simulink model "sysgenDWT"  (Simulink 7.0)
settings: Solver=ode45  StartTime=0.0  StopTime=4096+1024+100  RelTol=1e-3
PreLoadFcn:
  | xlrequire('imageData.mat'); xlrequire('PreLoadFcn');
PostLoadFcn:
  | open_system('sysgenDWT/Processor/Memory Controller','force'); pause(0.50); open_system('sysgenDWT');pause(0.50); close_system('sysgenDWT/Processor/Memory Controller');pause(0.50); close_system('sysgenDWT/Processor');
StopFcn:
  | xlrequire('StopFcn');
values from neighbouring files (symbols this model uses):
  b1Init = sysgenDWT_imageData( stride + dither )    [sysgenDWT_PreLoadFcn.m]
  b2Init = sysgenDWT_imageData( stride + not(dither) )    [sysgenDWT_PreLoadFcn.m]
libraries: xbsIndex_r4 x214, dspindex x4, dspmtrx3 x4, dspsnks4 x3, xbsCopyrightNotice_r4 x1, dspsrcs4 x1
(part 1 of 3)
settings Model: Creator=alexc  LastModifiedBy=douangp
settings DataIOCC: SignalLoggingName=sigsOut
settings OptimizationCC: BlockReduction=off  BooleanDataType=off  InlineInvariantSignals=on
settings DebuggingCC: SaveWithParameterizedLinksMsg=none  SignalResolutionControl=TryResolveAllWithWarning  SolverPrmCheckMsg=none  MultiTaskDSMMsg=warning  MultiTaskCondExecSysMsg=none  StrictBusMsg=None
settings HardwareCC: TargetUnknown=on
settings RTWCC: IncludeERTFirstTime=on
settings GRTTargetCC: TargetFcnLib=ansi_tfl_tmw.mat

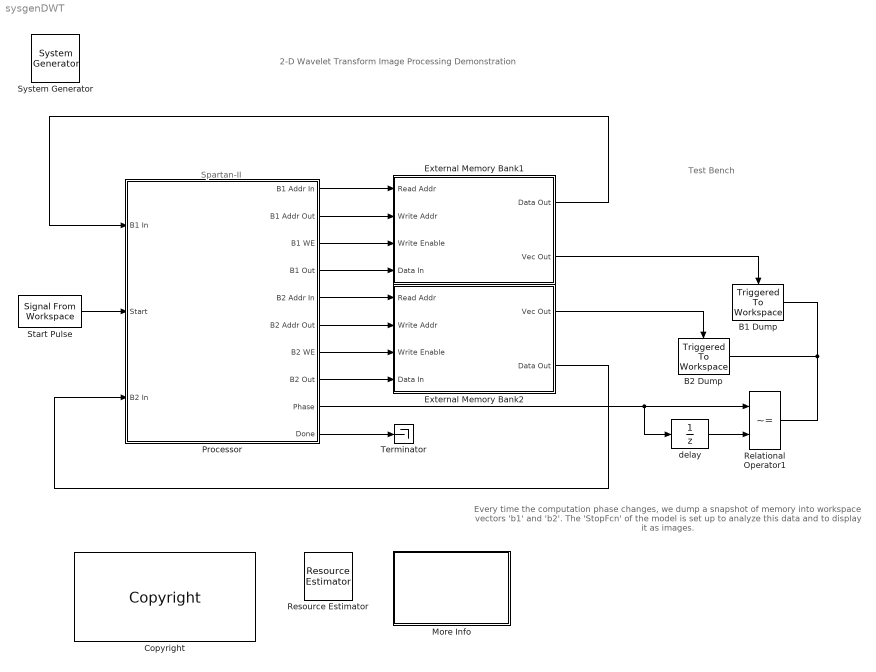
== system sysgenDWT ==
  note: Spartan-II
  note: Test
      |  Bench
  note: Every time the computation phase
      | changes, we dump a snapshot of
      | memory into workspace vectors  'b1'
      | and  'b2'.
      |
      | The 'StopFcn' of the model is set up
      | to analyze this data and to display
      | it as images.
  note: 2-D Wavelet Transform
      |  Image Processing Demonstration
  " System Generator" : xbsIndex_r4/ System Generator  Tag=genX  SystemSampleTime=-1  xilinxfamily=spartan3adsp  part=xc3sd3400a  speed=-4  package=fg676  synthesis_tool=XST  clock_wrapper=Clock Enables  directory=./netlist  testbench=off  simulink_period=1  sysclk_period=6  dcm_input_clock_period=100  incr_netlist=off  trim_vbits=Everywhere in SubSystem  dbl_ovrd=According to Block Masks  core_generation=Not Needed - Already Generated  run_coregen=off  deprecated_control=off  eval_field=0  block_type=sysgen
      settings: block_version=10.1.3
  B1 Dump : dspsnks4/Triggered To Workspace  Orientation=down  SystemSampleTime=-1  TriggerType=Falling edge  VariableName=b1  Buffer=1000
      settings: FixptAsFi=off
  B2 Dump : dspsnks4/Triggered To Workspace  Orientation=down  SystemSampleTime=-1  TriggerType=Falling edge  VariableName=b2  Buffer=1000
      settings: FixptAsFi=off
  Copyright : xbsCopyrightNotice_r4/Copyright  block_type=copyright
      settings: block_version=10.1.3
      settings: infoedit=|
      | Copyright(C) 2008 by  Xilinx, Inc. All rights reserved.<br>
      | <br>
      | This file contains proprietary, confidential information of Xilinx, Inc., is distributed under license
      | from Xilinx, Inc., and may be used, copied and/or disclosed only pursuant to the terms of a valid license
      | agreement with Xilinx, Inc. Xilinx hereby grants you a license to use this file solely for design,
      | simulation, implementation and creation of design files limited to Xilinx devices or technologies. Use
      | with non-Xilinx devices or technologies is expressly prohibited and immediately terminates your license
      | unless covered by a separate agreement.<br>
      | <br>
      | Xilinx is providing this design, code, or information "as-is" solely for use in developing programs and
      | solutions for Xilinx devices, with no obligation on the part of Xilinx to provide support. By providing
      | this design, code, or information as one possible implementation of this feature, application or standard,
      | Xilinx is making no representation that this implementation is free from any claims of infringement. You
      | are responsible for obtaining any rights you may require for your implementation. Xilinx expressly disclaims
      | any warranty whatsoever with respect to the adequacy of the implementation, including but not limited to any
      | warranties or representations that this implementation is free from claims of infringement, implied warranties
      | of merchantability or fitness for a particular purpose.<br>
      | <br>
      | Xilinx products are not intended for use in life support appliances, devices, or systems. Use in such
      | applications is expressly prohibited.<br>
      | <br>
      | Any modifications that are made to the Source Code are done at the user's sole risk and will be unsupported.<br>
      | <br>
      | This copyright and support notice must be retained as part of this text at all times.
      | (c) Copyright 1995-2008 Xilinx, Inc. All rights reserved.
  External Memory Bank1 : Subsystem  mask{depth=size (b2Init, 2), init_vec=b1Init}
      mask prompts: depth "Memory Depth"; init_vec "Initial Value"
  External Memory Bank2 : Subsystem  mask{depth=size (b2Init, 2), init_vec=b2Init}
      mask prompts: depth "Memory Depth"; init_vec "Initial Value"
  More Info : Subsystem
      mask Display: disp('Double click\n for\n more information.')
  Processor : Subsystem
  Relational Operator1 : RelationalOperator  Operator=~=  InputSameDT=on
  Resource Estimator : xbsIndex_r4/Resource Estimator  Tag=resEstTag  Slices=369  FFs=551  BRAMs=0  LUTs=422  IOBs=90  EBMs=0  TBUFs=0  xl_use_estimator_area=off  est_options=Estimate  xl_estimator_area=[369 551 0 422 90 0 0]  mrp_directory=e:/sg  simulink_period=1  block_type=resource_estimator
      settings: AttributesFormatString=Resource\nEstimator  block_version=10.1.3
  Start Pulse : dspsrcs4/Signal From Workspace  SystemSampleTime=-1  X=[ 0 0 0 1 0 0]  Ts=1  nsamps=1  OutputAfterFinalValue=Setting to zero  ignoreOrWarnInputAndFrameLengths=off
  Terminator : Terminator
  delay : UnitDelay  X0=-1
  wires:
  Processor/4(B1 Out) -> External Memory Bank1/4(Data In)
  Processor/3(B1 WE) -> External Memory Bank1/3(Write Enable)
  Processor/2(B1 Addr Out) -> External Memory Bank1/2(Write Addr)
  Processor/1(B1 Addr In) -> External Memory Bank1/1(Read Addr)
  Processor/5(B2 Addr In) -> External Memory Bank2/1(Read Addr)
  Processor/6(B2 Addr Out) -> External Memory Bank2/2(Write Addr)
  Processor/7(B2 WE) -> External Memory Bank2/3(Write Enable)
  Processor/8(B2 Out) -> External Memory Bank2/4(Data In)
  External Memory Bank1/1(Data Out) -> Processor/1(B1 In)
  External Memory Bank2/2(Data Out) -> Processor/3(B2 In)
  External Memory Bank2/1(Vec Out) -> B2 Dump/1
  External Memory Bank1/2(Vec Out) -> B1 Dump/1
  Processor/9(Phase) -> Relational Operator1/1, delay/1
  delay/1 -> Relational Operator1/2
  Relational Operator1/1 -> B1 Dump/Trigger, B2 Dump/Trigger
  Start Pulse/1 -> Processor/2(Start)
  Processor/10(Done) -> Terminator/1

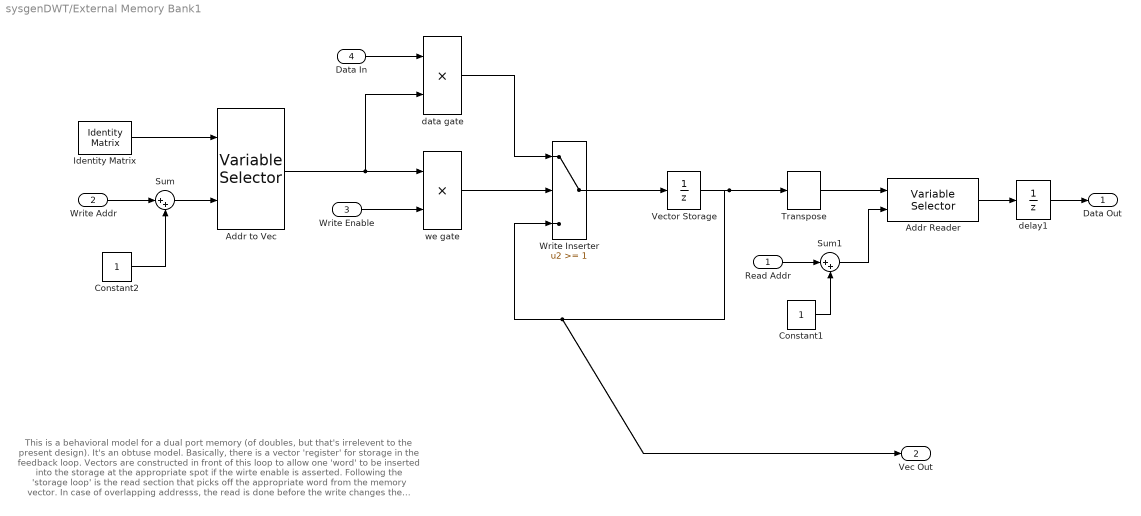
== system sysgenDWT/External Memory Bank1 ==
  note: This is a behavioral model for a dual port memory
      | (of doubles, but that's irrelevent to the present design).
      | It's an obtuse model.  Basically, there is a vector 'register'
      | for storage in the feedback loop. Vectors are constructed
      | in front of this loop to allow one 'word' to be inserted into the
      | storage  at the appropriate spot if the wirte enable is
      | asserted.  Following the 'storage loop' is the read section
      | that picks off the appropriate word from the memory vector.
      |
      | In case of overlapping addresss, the read is done before
      | the write changes the stored word.
      |
      | At every time step, the full contents of the memory are output
      | as a  vector of doubles.  This is a very handy  feature  for
      | analysis and debugging.
  Read Addr : Inport  OutDataType=sfix(16)  OutScaling=2^0
  Write Addr : Inport  Port=2  OutDataType=sfix(16)  OutScaling=2^0
  Write Enable : Inport  Port=3  OutDataType=sfix(16)  OutScaling=2^0
  Data In : Inport  Port=4  OutDataType=sfix(16)  OutScaling=2^0
  Addr Reader : dspindex/Variable Selector  NumInputs=1  rowsOrCols=Rows  IdxMode=Variable  Elements=[1 3]  ZerOneIdxMode=One-based  errmode=Generate Error  FillMode=on  FillValues=0
  Addr to Vec : dspindex/Variable Selector  NumInputs=1  rowsOrCols=Rows  IdxMode=Variable  Elements=[1 3]  ZerOneIdxMode=One-based  errmode=Clip Index  FillMode=on  FillValues=0
  Constant1 : Constant  OutDataType=sfix(16)  OutScaling=2^0
  Constant2 : Constant  OutDataType=sfix(16)  OutScaling=2^0
  Identity Matrix : dspmtrx3/Identity Matrix  Inherit=off  N=depth  Ts=1  dataType=double  isSigned=on  wordLen=16  udDataType=sfix(16)  fracBitsMode=Best precision  numFracBits=15
  Sum : Sum  Inputs=|++  OutDataType=sfix(16)  OutScaling=2^0  SaturateOnIntegerOverflow=on  InputSameDT=on
  Sum1 : Sum  Inputs=|++  OutDataType=sfix(16)  OutScaling=2^0  SaturateOnIntegerOverflow=on  InputSameDT=on
  Transpose : dspmtrx3/Transpose  SystemSampleTime=-1  Hermitian=off  overflowFlag=on
  Vector Storage : UnitDelay  X0=init_vec
  Write Inserter : Switch  Threshold=1  SaturateOnIntegerOverflow=on  InputSameDT=on
  data gate : Product  OutDataType=sfix(16)  OutScaling=2^0  SaturateOnIntegerOverflow=on  InputSameDT=on
  delay1 : UnitDelay
  we gate : Product  OutDataType=sfix(16)  OutScaling=2^0  SaturateOnIntegerOverflow=on  InputSameDT=on
  Data Out : Outport  OutDataType=sfix(16)  OutScaling=2^0
  Vec Out : Outport  Port=2  OutDataType=sfix(16)  OutScaling=2^0
  wires:
  Write Inserter/1 -> Vector Storage/1
  Addr Reader/1 -> delay1/1
  Addr to Vec/1 -> we gate/1, data gate/2
  Identity Matrix/1 -> Addr to Vec/1
  Write Enable/1 -> we gate/2
  Transpose/1 -> Addr Reader/1
  Data In/1 -> data gate/1
  we gate/1 -> Write Inserter/2
  data gate/1 -> Write Inserter/1
  Sum/1 -> Addr to Vec/2
  Write Addr/1 -> Sum/1
  Constant2/1 -> Sum/2
  Constant1/1 -> Sum1/2
  Sum1/1 -> Addr Reader/2
  delay1/1 -> Data Out/1
  Vector Storage/1 -> Transpose/1, Vec Out/1, Write Inserter/3
  Read Addr/1 -> Sum1/1

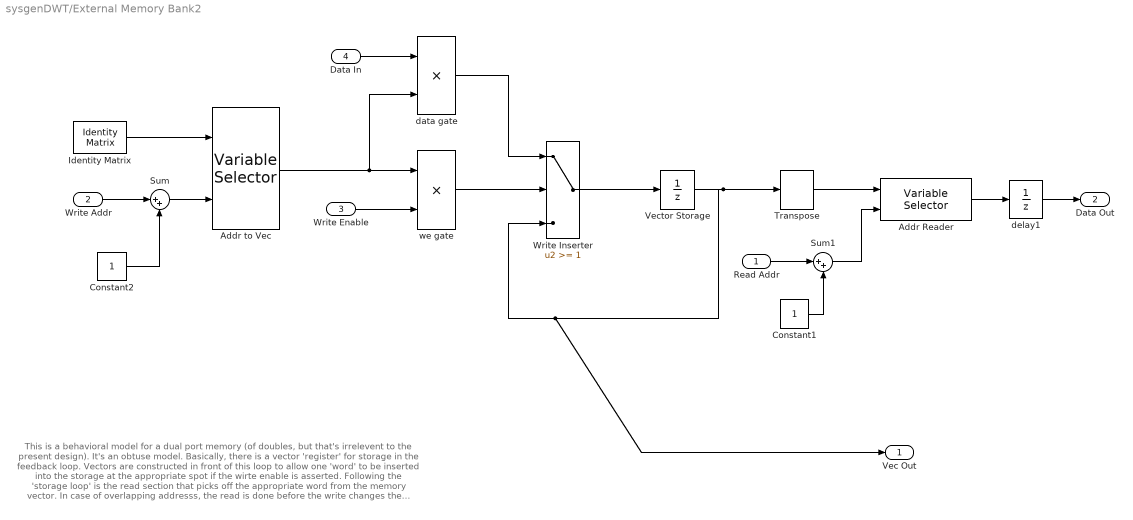
== system sysgenDWT/External Memory Bank2 ==
  note: This is a behavioral model for a dual port memory
      | (of doubles, but that's irrelevent to the present design).
      | It's an obtuse model.  Basically, there is a vector 'register'
      | for storage in the feedback loop. Vectors are constructed
      | in front of this loop to allow one 'word' to be inserted into the
      | storage  at the appropriate spot if the wirte enable is
      | asserted.  Following the 'storage loop' is the read section
      | that picks off the appropriate word from the memory vector.
      |
      | In case of overlapping addresss, the read is done before
      | the write changes the stored word.
      |
      | At every time step, the full contents of the memory are output
      | as a  vector of doubles.  This is a very handy  feature  for
      | analysis and debugging.
  Read Addr : Inport  OutDataType=sfix(16)  OutScaling=2^0
  Write Addr : Inport  Port=2  OutDataType=sfix(16)  OutScaling=2^0
  Write Enable : Inport  Port=3  OutDataType=sfix(16)  OutScaling=2^0
  Data In : Inport  Port=4  OutDataType=sfix(16)  OutScaling=2^0
  Addr Reader : dspindex/Variable Selector  NumInputs=1  rowsOrCols=Rows  IdxMode=Variable  Elements=[1 3]  ZerOneIdxMode=One-based  errmode=Clip Index  FillMode=on  FillValues=0
  Addr to Vec : dspindex/Variable Selector  NumInputs=1  rowsOrCols=Rows  IdxMode=Variable  Elements=[1 3]  ZerOneIdxMode=One-based  errmode=Clip Index  FillMode=on  FillValues=0
  Constant1 : Constant  OutDataType=sfix(16)  OutScaling=2^0
  Constant2 : Constant  OutDataType=sfix(16)  OutScaling=2^0
  Identity Matrix : dspmtrx3/Identity Matrix  Inherit=off  N=depth  Ts=1  dataType=double  isSigned=on  wordLen=16  udDataType=sfix(16)  fracBitsMode=Best precision  numFracBits=15
  Sum : Sum  Inputs=|++  OutDataType=sfix(16)  OutScaling=2^0  SaturateOnIntegerOverflow=on  InputSameDT=on
  Sum1 : Sum  Inputs=|++  OutDataType=sfix(16)  OutScaling=2^0  SaturateOnIntegerOverflow=on  InputSameDT=on
  Transpose : dspmtrx3/Transpose  SystemSampleTime=-1  Hermitian=off  overflowFlag=on
  Vector Storage : UnitDelay  X0=init_vec
  Write Inserter : Switch  Threshold=1  SaturateOnIntegerOverflow=on  InputSameDT=on
  data gate : Product  OutDataType=sfix(16)  OutScaling=2^0  SaturateOnIntegerOverflow=on  InputSameDT=on
  delay1 : UnitDelay
  we gate : Product  OutDataType=sfix(16)  OutScaling=2^0  SaturateOnIntegerOverflow=on  InputSameDT=on
  Vec Out : Outport  OutDataType=sfix(16)  OutScaling=2^0
  Data Out : Outport  Port=2  OutDataType=sfix(16)  OutScaling=2^0
  wires:
  Vector Storage/1 -> Transpose/1, Vec Out/1, Write Inserter/3
  delay1/1 -> Data Out/1
  Sum1/1 -> Addr Reader/2
  Read Addr/1 -> Sum1/1
  Constant1/1 -> Sum1/2
  Constant2/1 -> Sum/2
  Write Addr/1 -> Sum/1
  Sum/1 -> Addr to Vec/2
  data gate/1 -> Write Inserter/1
  we gate/1 -> Write Inserter/2
  Data In/1 -> data gate/1
  Transpose/1 -> Addr Reader/1
  Write Enable/1 -> we gate/2
  Identity Matrix/1 -> Addr to Vec/1
  Addr to Vec/1 -> data gate/2, we gate/1
  Addr Reader/1 -> delay1/1
  Write Inserter/1 -> Vector Storage/1

== system sysgenDWT/More Info ==
  note: The test bench for this wavelet design consists of a processor (built with the Xilinx Blockset for implementation in a Spartan-3A DSP
      | FPGA) and behavioral models for a pair of external, dual-port memories.  The two memories are initialized with the pixel values
      | of a grey-scale image.  The pixels from the initial image are interleaved into the two banks in a column first indexing strategy.
      | If the image contained a checkerboard of black and white pixels, then all of the black pixels will end up in the one bank, and all of
      | the white pixels in the other.  The processor includes a memory controller that schedules the reads and writes to memory, and
      | an image processing filter kernel that computes the 2D DWT decomposition of the image.  The processor has been configured
      | to compute two levels of decomposition on a 64 x 64 pixel image. The computation is done "in place" in the single image memory
      | space, and the initial pixel ordering is preserved throughout.
      |
      | The design occupies 347 LUTs , 496 Slice Registers  of an xc3sd3400a-4 and runs at 166 MHz
      | (processing 320 MPixels per second) in a low-cost, high-volume, Spartan-3A DSP device. (10.1.3 software, VHDL synthesized with XST).
      |
      | A full color version of the design would easily fit in the same part as only the DWT datapath would require replication (the memoy
      | control could remain unchanged).
  note: 2-D Wavelet Transform Image Processing Demonstration

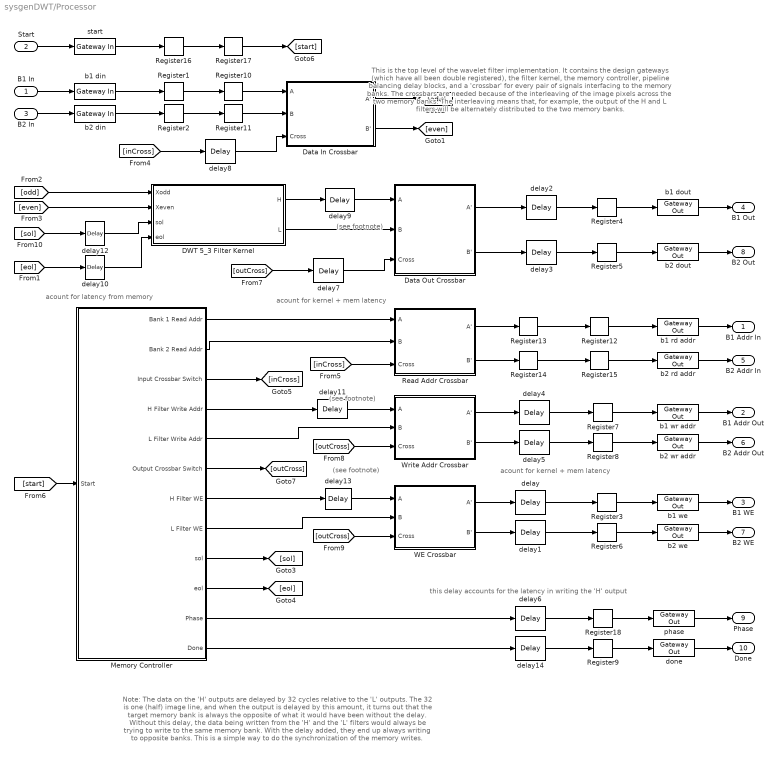
== system sysgenDWT/Processor ==
  note: This is the top level of the wavelet filter implementation.
      | It contains the design gateways (which have all been double
      | registered),  the filter kernel, the memory controller, pipeline
      | balancing delay blocks, and a 'crossbar' for every pair of signals
      | interfacing to the memory banks.  The crossbars are needed
      | because of the interleaving of the image pixels across the two
      | memory banks.  The interleaving means that, for example,
      | the output of the H and L filters will be alternately distributed
      | to the two memory banks.
  note: (see footnote)
  note: (see footnote)
  note: (see footnote)
  note: Note: The data on the 'H' outputs are delayed by 32 cycles relative to the 'L' outputs.
      | The 32 is one (half) image line, and when the output is delayed by this amount, it
      | turns out that the target memory bank is always the opposite of what it would have
      | been without the delay.  Without this delay, the data being written from the 'H' and
      | the 'L' filters would always be trying to write to the same memory bank.  With the
      | delay added, they end up always writing to opposite banks.  This is a simple way
      | to do the synchronization of the memory writes.
  note: this delay accounts for
      | the latency in writing the 'H' output
  note: acount for latency from memory
  note: acount for kernel + mem latency
  note: acount for kernel + mem latency
  B1 In : Inport  OutDataType=sfix(16)  OutScaling=2^0
  Start : Inport  Port=2  OutDataType=sfix(16)  OutScaling=2^0
  B2 In : Inport  Port=3  OutDataType=sfix(16)  OutScaling=2^0
  DWT 5_3 Filter Kernel : Subsystem
  Data In Crossbar : Subsystem
  Data Out Crossbar : Subsystem
  Memory Controller : Subsystem  mask{N=6, M=6}
      mask prompts: N "Log Base 2 of Image Width"; M "Log Base 2 of Image Height"
  Read Addr Crossbar : Subsystem
  Register{1..18} (18 alike) : xbsIndex_r4/Register  init=0  rst=off  en=off  dbl_ovrd=off  block_type=register
      Register1 settings: xl_area=[5 10 0 0 0 0 0]  block_version=VER_STRING_GOES_HERE
      Register10 settings: xl_area=[5 10 0 0 0 0 0]  block_version=VER_STRING_GOES_HERE
      Register11 settings: xl_area=[5 10 0 0 0 0 0]  block_version=VER_STRING_GOES_HERE
      Register12 settings: xl_area=[6 11 0 0 0 0 0]  block_version=VER_STRING_GOES_HERE
      Register13 settings: xl_area=[6 11 0 0 0 0 0]  block_version=VER_STRING_GOES_HERE
      Register14 settings: xl_area=[6 11 0 0 0 0 0]  block_version=VER_STRING_GOES_HERE
      Register15 settings: xl_area=[6 11 0 0 0 0 0]  block_version=VER_STRING_GOES_HERE
      Register16 settings: xl_area=[1 1 0 0 0 0 0]  block_version=VER_STRING_GOES_HERE
      Register17 settings: xl_area=[1 1 0 0 0 0 0]  block_version=VER_STRING_GOES_HERE
      Register18 settings: xl_area=[1 2 0 0 0 0 0]  block_version=VER_STRING_GOES_HERE
      Register2 settings: xl_area=[5 10 0 0 0 0 0]  block_version=VER_STRING_GOES_HERE
      Register3 settings: xl_area=[1 1 0 0 0 0 0]  block_version=VER_STRING_GOES_HERE
      Register4 settings: xl_area=[5 10 0 0 0 0 0]  block_version=VER_STRING_GOES_HERE
      Register5 settings: xl_area=[5 10 0 0 0 0 0]  block_version=VER_STRING_GOES_HERE
      Register6 settings: xl_area=[1 1 0 0 0 0 0]  block_version=VER_STRING_GOES_HERE
      Register7 settings: xl_area=[6 11 0 0 0 0 0]  block_version=VER_STRING_GOES_HERE
      Register8 settings: xl_area=[6 11 0 0 0 0 0]  block_version=VER_STRING_GOES_HERE
      Register9 settings: xl_area=[1 1 0 0 0 0 0]  block_version=VER_STRING_GOES_HERE
  WE Crossbar : Subsystem
  Write Addr Crossbar : Subsystem
  b1 din : xbsIndex_r4/Gateway In  arith_type="Signed  (2's comp)"  n_bits=10  bin_pt=0  quantization="Round  (unbiased: +/- Inf)"  overflow=Saturate  period=1  dbl_ovrd=off  timing_constraint=None  locs_specified=off  LOCs={}  block_type=gatewayin
      settings: infoedit="Gateway in block.  Converts inputs of type Simulink integer, double and fixed point to  Xilinx fixed point type.<P><P>Hardware notes:  In hardware these blocks become top level input ports."  xl_area=[0 0 0 0 10 0 0]  block_version=VER_STRING_GOES_HERE
  b1 dout : xbsIndex_r4/Gateway Out  hdl_port=on  timing_constraint=None  locs_specified=off  LOCs={}  block_type=gatewayout
      settings: infoedit="Gateway out block.  Converts Xilinx fixed point inputs into ouputs of type Simulink integer, double, or fixed point.<P><P>Hardware notes:  In hardware these blocks become top level output ports or are discarded, depending on how they are configured."  xl_area=[0 0 0 0 10 0 0]  block_version=VER_STRING_GOES_HERE
  b1 rd addr : xbsIndex_r4/Gateway Out  hdl_port=on  timing_constraint=None  locs_specified=off  LOCs={}  block_type=gatewayout
      settings: infoedit="Gateway out block.  Converts Xilinx fixed point inputs into ouputs of type Simulink integer, double, or fixed point.<P><P>Hardware notes:  In hardware these blocks become top level output ports or are discarded, depending on how they are configured."  xl_area=[0 0 0 0 11 0 0]  block_version=VER_STRING_GOES_HERE
  b1 we : xbsIndex_r4/Gateway Out  hdl_port=on  timing_constraint=None  locs_specified=off  LOCs={}  block_type=gatewayout
      settings: infoedit="Gateway out block.  Converts Xilinx fixed point inputs into ouputs of type Simulink integer, double, or fixed point.<P><P>Hardware notes:  In hardware these blocks become top level output ports or are discarded, depending on how they are configured."  xl_area=[0 0 0 0 1 0 0]  block_version=VER_STRING_GOES_HERE
  b1 wr addr : xbsIndex_r4/Gateway Out  hdl_port=on  timing_constraint=None  locs_specified=off  LOCs={}  block_type=gatewayout
      settings: infoedit="Gateway out block.  Converts Xilinx fixed point inputs into ouputs of type Simulink integer, double, or fixed point.<P><P>Hardware notes:  In hardware these blocks become top level output ports or are discarded, depending on how they are configured."  xl_area=[0 0 0 0 11 0 0]  block_version=VER_STRING_GOES_HERE
  b2 din : xbsIndex_r4/Gateway In  arith_type="Signed  (2's comp)"  n_bits=10  bin_pt=0  quantization="Round  (unbiased: +/- Inf)"  overflow=Saturate  period=1  dbl_ovrd=off  timing_constraint=None  locs_specified=off  LOCs={}  block_type=gatewayin
      settings: infoedit="Gateway in block.  Converts inputs of type Simulink integer, double and fixed point to  Xilinx fixed point type.<P><P>Hardware notes:  In hardware these blocks become top level input ports."  xl_area=[0 0 0 0 10 0 0]  block_version=VER_STRING_GOES_HERE
  b2 dout : xbsIndex_r4/Gateway Out  hdl_port=on  timing_constraint=None  locs_specified=off  LOCs={}  block_type=gatewayout
      settings: infoedit="Gateway out block.  Converts Xilinx fixed point inputs into ouputs of type Simulink integer, double, or fixed point.<P><P>Hardware notes:  In hardware these blocks become top level output ports or are discarded, depending on how they are configured."  xl_area=[0 0 0 0 10 0 0]  block_version=VER_STRING_GOES_HERE
  b2 rd addr : xbsIndex_r4/Gateway Out  hdl_port=on  timing_constraint=None  locs_specified=off  LOCs={}  block_type=gatewayout
      settings: infoedit="Gateway out block.  Converts Xilinx fixed point inputs into ouputs of type Simulink integer, double, or fixed point.<P><P>Hardware notes:  In hardware these blocks become top level output ports or are discarded, depending on how they are configured."  xl_area=[0 0 0 0 11 0 0]  block_version=VER_STRING_GOES_HERE
  b2 we : xbsIndex_r4/Gateway Out  hdl_port=on  timing_constraint=None  locs_specified=off  LOCs={}  block_type=gatewayout
      settings: infoedit="Gateway out block.  Converts Xilinx fixed point inputs into ouputs of type Simulink integer, double, or fixed point.<P><P>Hardware notes:  In hardware these blocks become top level output ports or are discarded, depending on how they are configured."  xl_area=[0 0 0 0 1 0 0]  block_version=VER_STRING_GOES_HERE
  b2 wr addr : xbsIndex_r4/Gateway Out  hdl_port=on  timing_constraint=None  locs_specified=off  LOCs={}  block_type=gatewayout
      settings: infoedit="Gateway out block.  Converts Xilinx fixed point inputs into ouputs of type Simulink integer, double, or fixed point.<P><P>Hardware notes:  In hardware these blocks become top level output ports or are discarded, depending on how they are configured."  xl_area=[0 0 0 0 11 0 0]  block_version=VER_STRING_GOES_HERE
  delay{,1,4..5} (4 alike) : xbsIndex_r4/Delay  en=off  latency=15  dbl_ovrd=off  reg_retiming=off  block_type=delay
      delay settings: infoedit="Delay line having  configurable length.<P><P>Hardware notes: A delay line is a chain, each link of which is an SRL16 followed by a flip-flop. If register retiming is enabled, the delay line is a chain of flip-flops."  xl_area=[1 1 0 1 0 0 0]  block_version=VER_STRING_GOES_HERE
      delay1 settings: infoedit="Delay line having  configurable length.<P><P>Hardware notes: A delay line is a chain, each link of which is an SRL16 followed by a flip-flop. If register retiming is enabled, the delay line is a chain of flip-flops."  xl_area=[1 1 0 1 0 0 0]  block_version=VER_STRING_GOES_HERE
      delay4 settings: infoedit="Delay line having  configurable length.<P><P>Hardware notes: A delay line is a chain, each link of which is an SRL16 followed by a flip-flop. If register retiming is enabled, the delay line is a chain of flip-flops."  xl_area=[6 11 0 11 0 0 0]  block_version=VER_STRING_GOES_HERE
      delay5 settings: infoedit="Delay line having  configurable length.<P><P>Hardware notes: A delay line is a chain, each link of which is an SRL16 followed by a flip-flop. If register retiming is enabled, the delay line is a chain of flip-flops."  xl_area=[6 11 0 11 0 0 0]  block_version=VER_STRING_GOES_HERE
  delay10 : xbsIndex_r4/Delay  en=off  latency=6  dbl_ovrd=off  reg_retiming=off  block_type=delay
      settings: infoedit="Delay line having  configurable length.<P><P>Hardware notes: A delay line is a chain, each link of which is an SRL16 followed by a flip-flop. If register retiming is enabled, the delay line is a chain of flip-flops."  xl_area=[1 1 0 1 0 0 0]  block_version=VER_STRING_GOES_HERE
  delay11 : xbsIndex_r4/Delay  en=off  latency=32  dbl_ovrd=off  reg_retiming=off  block_type=delay
      settings: infoedit="Delay line having  configurable length.<P><P>Hardware notes: A delay line is a chain, each link of which is an SRL16 followed by a flip-flop. If register retiming is enabled, the delay line is a chain of flip-flops."  xl_area=[12 22 0 22 0 0 0]  block_version=VER_STRING_GOES_HERE
  delay12 : xbsIndex_r4/Delay  en=off  latency=6  dbl_ovrd=off  reg_retiming=off  block_type=delay
      settings: infoedit="Delay line having  configurable length.<P><P>Hardware notes: A delay line is a chain, each link of which is an SRL16 followed by a flip-flop. If register retiming is enabled, the delay line is a chain of flip-flops."  xl_area=[1 1 0 1 0 0 0]  block_version=VER_STRING_GOES_HERE
  delay13 : xbsIndex_r4/Delay  en=off  latency=32  dbl_ovrd=off  reg_retiming=off  block_type=delay
      settings: infoedit="Delay line having  configurable length.<P><P>Hardware notes: A delay line is a chain, each link of which is an SRL16 followed by a flip-flop. If register retiming is enabled, the delay line is a chain of flip-flops."  xl_area=[2 2 0 2 0 0 0]  block_version=VER_STRING_GOES_HERE
  delay14 : xbsIndex_r4/Delay  en=off  latency=32+15  dbl_ovrd=off  reg_retiming=off  block_type=delay
      settings: infoedit="Delay line having  configurable length.<P><P>Hardware notes: A delay line is a chain, each link of which is an SRL16 followed by a flip-flop. If register retiming is enabled, the delay line is a chain of flip-flops."  xl_area=[3 3 0 3 0 0 0]  block_version=VER_STRING_GOES_HERE
  delay2 : xbsIndex_r4/Delay  en=off  latency=1  dbl_ovrd=off  reg_retiming=off  block_type=delay
      settings: infoedit="Delay line having  configurable length.<P><P>Hardware notes: A delay line is a chain, each link of which is an SRL16 followed by a flip-flop. If register retiming is enabled, the delay line is a chain of flip-flops."  xl_area=[5 10 0 0 0 0 0]  block_version=VER_STRING_GOES_HERE
  delay3 : xbsIndex_r4/Delay  en=off  latency=1  dbl_ovrd=off  reg_retiming=off  block_type=delay
      settings: infoedit="Delay line having  configurable length.<P><P>Hardware notes: A delay line is a chain, each link of which is an SRL16 followed by a flip-flop. If register retiming is enabled, the delay line is a chain of flip-flops."  xl_area=[5 10 0 0 0 0 0]  block_version=VER_STRING_GOES_HERE
  delay6 : xbsIndex_r4/Delay  en=off  latency=32+15  dbl_ovrd=off  reg_retiming=off  block_type=delay
      settings: infoedit="Delay line having  configurable length.<P><P>Hardware notes: A delay line is a chain, each link of which is an SRL16 followed by a flip-flop. If register retiming is enabled, the delay line is a chain of flip-flops."  xl_area=[3 6 0 6 0 0 0]  block_version=VER_STRING_GOES_HERE
  delay7 : xbsIndex_r4/Delay  en=off  latency=14  dbl_ovrd=off  reg_retiming=off  block_type=delay
      settings: infoedit="Delay line having  configurable length.<P><P>Hardware notes: A delay line is a chain, each link of which is an SRL16 followed by a flip-flop. If register retiming is enabled, the delay line is a chain of flip-flops."  xl_area=[1 1 0 1 0 0 0]  block_version=VER_STRING_GOES_HERE
  delay8 : xbsIndex_r4/Delay  en=off  latency=6  dbl_ovrd=off  reg_retiming=off  block_type=delay
      settings: infoedit="Delay line having  configurable length.<P><P>Hardware notes: A delay line is a chain, each link of which is an SRL16 followed by a flip-flop. If register retiming is enabled, the delay line is a chain of flip-flops."  xl_area=[1 1 0 1 0 0 0]  block_version=VER_STRING_GOES_HERE
  delay9 : xbsIndex_r4/Delay  en=off  latency=32  dbl_ovrd=off  reg_retiming=off  block_type=delay
      settings: infoedit="Delay line having  configurable length.<P><P>Hardware notes: A delay line is a chain, each link of which is an SRL16 followed by a flip-flop. If register retiming is enabled, the delay line is a chain of flip-flops."  xl_area=[10 20 0 20 0 0 0]  block_version=VER_STRING_GOES_HERE
  done : xbsIndex_r4/Gateway Out  hdl_port=on  timing_constraint=None  locs_specified=off  LOCs={}  block_type=gatewayout
      settings: infoedit="Gateway out block.  Converts Xilinx fixed point inputs into ouputs of type Simulink integer, double, or fixed point.<P><P>Hardware notes:  In hardware these blocks become top level output ports or are discarded, depending on how they are configured."  xl_area=[0 0 0 0 1 0 0]  block_version=VER_STRING_GOES_HERE
  phase : xbsIndex_r4/Gateway Out  hdl_port=on  timing_constraint=None  locs_specified=off  LOCs={}  block_type=gatewayout
      settings: infoedit="Gateway out block.  Converts Xilinx fixed point inputs into ouputs of type Simulink integer, double, or fixed point.<P><P>Hardware notes:  In hardware these blocks become top level output ports or are discarded, depending on how they are configured."  xl_area=[0 0 0 0 2 0 0]  block_version=VER_STRING_GOES_HERE
  start : xbsIndex_r4/Gateway In  arith_type=Boolean  n_bits=1  bin_pt=0  quantization="Round  (unbiased: +/- Inf)"  overflow=Saturate  period=1  dbl_ovrd=off  timing_constraint=None  locs_specified=off  LOCs={}  block_type=gatewayin
      settings: infoedit="Gateway in block.  Converts inputs of type Simulink integer, double and fixed point to  Xilinx fixed point type.<P><P>Hardware notes:  In hardware these blocks become top level input ports."  xl_area=[0 0 0 0 1 0 0]  block_version=VER_STRING_GOES_HERE
  B1 Addr In : Outport  OutDataType=sfix(16)  OutScaling=2^0
  B1 Addr Out : Outport  Port=2  OutDataType=sfix(16)  OutScaling=2^0
  B1 WE : Outport  Port=3  OutDataType=sfix(16)  OutScaling=2^0
  B1 Out : Outport  Port=4  OutDataType=sfix(16)  OutScaling=2^0
  B2 Addr In : Outport  Port=5  OutDataType=sfix(16)  OutScaling=2^0
  B2 Addr Out : Outport  Port=6  OutDataType=sfix(16)  OutScaling=2^0
  B2 WE : Outport  Port=7  OutDataType=sfix(16)  OutScaling=2^0
  B2 Out : Outport  Port=8  OutDataType=sfix(16)  OutScaling=2^0
  Phase : Outport  Port=9  OutDataType=sfix(16)  OutScaling=2^0
  Done : Outport  Port=10  OutDataType=sfix(16)  OutScaling=2^0
  wires:
  b1 din/1 -> Register1/1
  b2 din/1 -> Register2/1
  [sol] -> delay12/1
  [eol] -> delay10/1
  [odd] -> DWT 5_3 Filter Kernel/1(Xodd)
  [even] -> DWT 5_3 Filter Kernel/2(Xeven)
  Register1/1 -> Register10/1
  Register2/1 -> Register11/1
  Memory Controller/5(L Filter Write Addr) -> Write Addr Crossbar/2(B)
  Memory Controller/4(H Filter Write Addr) -> delay11/1
  Memory Controller/11(Phase) -> delay6/1
  Memory Controller/9(sol) -> [sol]
  Memory Controller/10(eol) -> [eol]
  Write Addr Crossbar/1(A') -> delay4/1
  Write Addr Crossbar/2(B') -> delay5/1
  DWT 5_3 Filter Kernel/1(H) -> delay9/1
  DWT 5_3 Filter Kernel/2(L) -> Data Out Crossbar/2(B)
  Data Out Crossbar/1(A') -> delay2/1
  Data Out Crossbar/2(B') -> delay3/1
  Register4/1 -> b1 dout/1
  Register5/1 -> b2 dout/1
  b2 rd addr/1 -> B2 Addr In/1
  b1 wr addr/1 -> B1 Addr Out/1
  b2 wr addr/1 -> B2 Addr Out/1
  B1 In/1 -> b1 din/1
  B2 In/1 -> b2 din/1
  b1 dout/1 -> B1 Out/1
  b2 dout/1 -> B2 Out/1
  b1 we/1 -> B1 WE/1
  b2 we/1 -> B2 WE/1
  delay2/1 -> Register4/1
  delay3/1 -> Register5/1
  delay5/1 -> Register8/1
  delay4/1 -> Register7/1
  Register7/1 -> b1 wr addr/1
  Register8/1 -> b2 wr addr/1
  phase/1 -> Phase/1
  Data In Crossbar/1(A') -> [odd]
  Data In Crossbar/2(B') -> [even]
  Memory Controller/3(Input Crossbar Switch) -> [inCross]
  Read Addr Crossbar/1(A') -> Register13/1
  Read Addr Crossbar/2(B') -> Register14/1
  Memory Controller/2(Bank 2 Read Addr) -> Read Addr Crossbar/2(B)
  Memory Controller/1(Bank 1 Read Addr) -> Read Addr Crossbar/1(A)
  delay6/1 -> Register18/1
  delay7/1 -> Data Out Crossbar/3(Cross)
  delay8/1 -> Data In Crossbar/3(Cross)
  [inCross] -> delay8/1
  [inCross] -> Read Addr Crossbar/3(Cross)
  delay10/1 -> DWT 5_3 Filter Kernel/4(eol)
  delay12/1 -> DWT 5_3 Filter Kernel/3(sol)
  delay9/1 -> Data Out Crossbar/1(A)
  delay11/1 -> Write Addr Crossbar/1(A)
  delay1/1 -> Register6/1
  delay/1 -> Register3/1
  WE Crossbar/2(B') -> delay1/1
  WE Crossbar/1(A') -> delay/1
  delay13/1 -> WE Crossbar/1(A)
  Register3/1 -> b1 we/1
  Register6/1 -> b2 we/1
  Register10/1 -> Data In Crossbar/1(A)
  Register11/1 -> Data In Crossbar/2(B)
  Register12/1 -> b1 rd addr/1
  Register13/1 -> Register12/1
  Register14/1 -> Register15/1
  Register15/1 -> b2 rd addr/1
  Start/1 -> start/1
  start/1 -> Register16/1
  Register16/1 -> Register17/1
  Register17/1 -> [start]
  [start] -> Memory Controller/1(Start)
  Memory Controller/6(Output Crossbar Switch) -> [outCross]
  [outCross] -> delay7/1
  [outCross] -> Write Addr Crossbar/3(Cross)
  [outCross] -> WE Crossbar/3(Cross)
  done/1 -> Done/1
  delay14/1 -> Register9/1
  Register9/1 -> done/1
  Register18/1 -> phase/1
  Memory Controller/12(Done) -> delay14/1
  b1 rd addr/1 -> B1 Addr In/1
  Memory Controller/7(H Filter WE) -> delay13/1
  Memory Controller/8(L Filter WE) -> WE Crossbar/2(B)

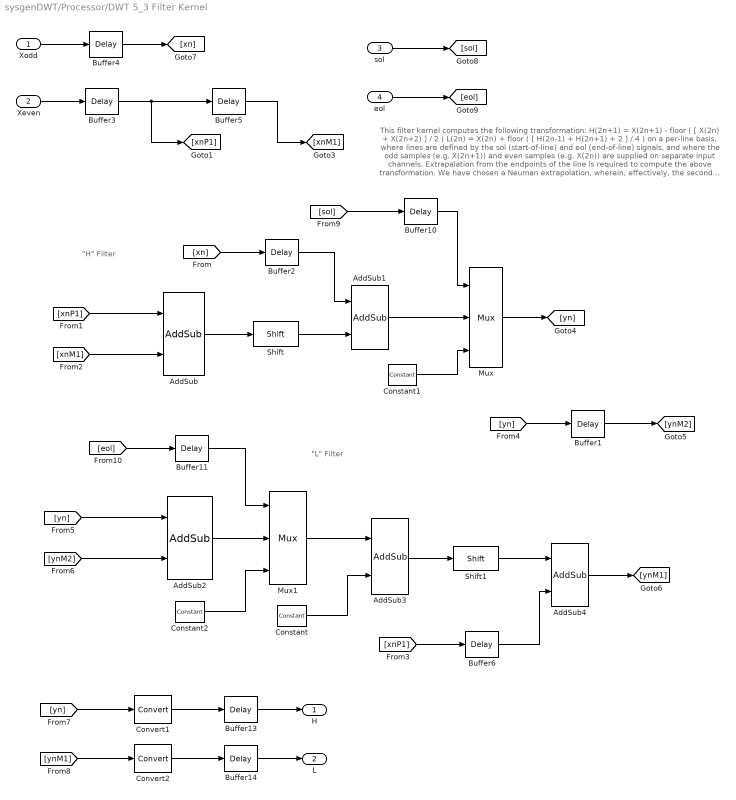
== system sysgenDWT/Processor/DWT 5_3 Filter Kernel ==
  note: This filter kernel computes the following transformation:
      |
      |    H(2n+1) = X(2n+1) - floor ( [ X(2n) + X(2n+2) ] / 2 )
      |    L(2n)      =  X(2n)  + floor ( [ H(2n-1) + H(2n+1) + 2 ] / 4 )
      |
      | on a per-line basis, where lines are defined by the sol
      | (start-of-line) and eol (end-of-line) signals, and where
      | the odd samples (e.g. X(2n+1)) and even samples
      | (e.g. X(2n)) are supplied on separate input channels.
      |
      | Extrapalation from the endpoints of the line is required
      | to compute the above transformation.  We have chosen
      | a Neuman extrapolation, wherein, effectively, the second
      | derivative of the data becomes zero at the endpoint and
      | the data is inflected.  Thus, with x(1) being an endpoint,
      | we construct:
      |    X(0) = X(1) - [ X(2) - X(1) ]        and
      |    X(-1) = X(1) - 2 [ X(3) - X(1) ]
      |
      | This extrapolation scheme becomes very simple in
      | the hardware implementation, adding only the two muxes
      | appearing below.
  note: "H" Filter
  note: "L" Filter
  Xodd : Inport  OutDataType=sfix(16)  OutScaling=2^0
  Xeven : Inport  Port=2  OutDataType=sfix(16)  OutScaling=2^0
  sol : Inport  Port=3  OutDataType=sfix(16)  OutScaling=2^0
  eol : Inport  Port=4  OutDataType=sfix(16)  OutScaling=2^0
  AddSub{,2..4} (4 alike) : xbsIndex_r4/AddSub  mode=Addition  use_carryin=off  use_carryout=off  en=off  latency=1  precision=Full  arith_type=Unsigned  n_bits=8  bin_pt=2  quantization=Truncate  overflow=Wrap  dbl_ovrd=off  use_behavioral_HDL=on  pipelined=off  use_rpm=off  hw_selection=Fabric  block_type=addsub
      AddSub settings: xl_area=[6 11 0 10 0 0 0]  block_version=VER_STRING_GOES_HERE
      AddSub2 settings: xl_area=[6 12 0 11 0 0 0]  block_version=VER_STRING_GOES_HERE
      AddSub3 settings: xl_area=[7 13 0 8 0 0 0]  block_version=VER_STRING_GOES_HERE
      AddSub4 settings: xl_area=[6 12 0 11 0 0 0]  block_version=VER_STRING_GOES_HERE
  AddSub1 : xbsIndex_r4/AddSub  mode=Subtraction  use_carryin=off  use_carryout=off  en=off  latency=1  precision=Full  arith_type=Unsigned  n_bits=8  bin_pt=2  quantization=Truncate  overflow=Wrap  dbl_ovrd=off  use_behavioral_HDL=on  pipelined=off  use_rpm=off  hw_selection=Fabric  block_type=addsub
      settings: xl_area=[6 11 0 10 0 0 0]  block_version=VER_STRING_GOES_HERE
  Buffer{1..5,14} (6 alike) : xbsIndex_r4/Delay  en=off  latency=1  dbl_ovrd=off  reg_retiming=off  block_type=delay
      Buffer1 settings: infoedit="Delay line having  configurable length.<P><P>Hardware notes: A delay line is a chain, each link of which is an SRL16 followed by a flip-flop. If register retiming is enabled, the delay line is a chain of flip-flops."  xl_area=[6 11 0 0 0 0 0]  block_version=VER_STRING_GOES_HERE
      Buffer14 settings: infoedit="Delay line having  configurable length.<P><P>Hardware notes: A delay line is a chain, each link of which is an SRL16 followed by a flip-flop. If register retiming is enabled, the delay line is a chain of flip-flops."  xl_area=[5 10 0 0 0 0 0]  block_version=VER_STRING_GOES_HERE
      Buffer2 settings: infoedit="Delay line having  configurable length.<P><P>Hardware notes: A delay line is a chain, each link of which is an SRL16 followed by a flip-flop. If register retiming is enabled, the delay line is a chain of flip-flops."  xl_area=[5 10 0 0 0 0 0]  block_version=VER_STRING_GOES_HERE
      Buffer3 settings: infoedit="Delay line having  configurable length.<P><P>Hardware notes: A delay line is a chain, each link of which is an SRL16 followed by a flip-flop. If register retiming is enabled, the delay line is a chain of flip-flops."  xl_area=[5 10 0 0 0 0 0]  block_version=VER_STRING_GOES_HERE
      Buffer4 settings: infoedit="Delay line having  configurable length.<P><P>Hardware notes: A delay line is a chain, each link of which is an SRL16 followed by a flip-flop. If register retiming is enabled, the delay line is a chain of flip-flops."  xl_area=[5 10 0 0 0 0 0]  block_version=VER_STRING_GOES_HERE
      Buffer5 settings: infoedit="Delay line having  configurable length.<P><P>Hardware notes: A delay line is a chain, each link of which is an SRL16 followed by a flip-flop. If register retiming is enabled, the delay line is a chain of flip-flops."  xl_area=[5 10 0 0 0 0 0]  block_version=VER_STRING_GOES_HERE
  Buffer10 : xbsIndex_r4/Delay  en=off  latency=3  dbl_ovrd=off  reg_retiming=off  block_type=delay
      settings: infoedit="Delay line having  configurable length.<P><P>Hardware notes: A delay line is a chain, each link of which is an SRL16 followed by a flip-flop. If register retiming is enabled, the delay line is a chain of flip-flops."  xl_area=[1 1 0 1 0 0 0]  block_version=VER_STRING_GOES_HERE
  Buffer11 : xbsIndex_r4/Delay  en=off  latency=7  dbl_ovrd=off  reg_retiming=off  block_type=delay
      settings: infoedit="Delay line having  configurable length.<P><P>Hardware notes: A delay line is a chain, each link of which is an SRL16 followed by a flip-flop. If register retiming is enabled, the delay line is a chain of flip-flops."  xl_area=[1 1 0 1 0 0 0]  block_version=VER_STRING_GOES_HERE
  Buffer13 : xbsIndex_r4/Delay  en=off  latency=6  dbl_ovrd=off  reg_retiming=off  block_type=delay
      settings: infoedit="Delay line having  configurable length.<P><P>Hardware notes: A delay line is a chain, each link of which is an SRL16 followed by a flip-flop. If register retiming is enabled, the delay line is a chain of flip-flops."  xl_area=[5 10 0 10 0 0 0]  block_version=VER_STRING_GOES_HERE
  Buffer6 : xbsIndex_r4/Delay  en=off  latency=5  dbl_ovrd=off  reg_retiming=off  block_type=delay
      settings: infoedit="Delay line having  configurable length.<P><P>Hardware notes: A delay line is a chain, each link of which is an SRL16 followed by a flip-flop. If register retiming is enabled, the delay line is a chain of flip-flops."  xl_area=[5 10 0 10 0 0 0]  block_version=VER_STRING_GOES_HERE
  Constant : xbsIndex_r4/Constant  arith_type=Unsigned  const=2  n_bits=2  bin_pt=0  explicit_period=off  period=1  equ=P=C  opselect=C  inp2=PCIN>>17  opr=+  inp1=P  carry=CIN  dbl_ovrd=off  block_type=constant
      settings: block_version=VER_STRING_GOES_HERE
  Constant1 : xbsIndex_r4/Constant  arith_type=Signed (2's comp)  const=0  n_bits=11  bin_pt=0  explicit_period=off  period=1  equ=P=C  opselect=C  inp2=PCIN>>17  opr=+  inp1=P  carry=CIN  dbl_ovrd=off  block_type=constant
      settings: block_version=VER_STRING_GOES_HERE
  Constant2 : xbsIndex_r4/Constant  arith_type=Signed (2's comp)  const=0  n_bits=12  bin_pt=0  explicit_period=off  period=1  equ=P=C  opselect=C  inp2=PCIN>>17  opr=+  inp1=P  carry=CIN  dbl_ovrd=off  block_type=constant
      settings: block_version=VER_STRING_GOES_HERE
  Convert1 : xbsIndex_r4/Convert  arith_type="Signed  (2's comp)"  n_bits=10  bin_pt=0  quantization="Round  (unbiased: +/- Inf)"  overflow=Saturate  latency=0  dbl_ovrd=off  pipeline=off  block_type=convert
      settings: infoedit=The input is presented at the output after quantization and overflow effects.<P><P>Hardware notes: Additional hardware is used when rounding or saturation is selected and output width is less than the input width.  xl_area=[5 0 0 10 0 0 0]  block_version=VER_STRING_GOES_HERE
  Convert2 : xbsIndex_r4/Convert  arith_type="Signed  (2's comp)"  n_bits=10  bin_pt=0  quantization="Round  (unbiased: +/- Inf)"  overflow=Saturate  latency=0  dbl_ovrd=off  pipeline=off  block_type=convert
      settings: infoedit=The input is presented at the output after quantization and overflow effects.<P><P>Hardware notes: Additional hardware is used when rounding or saturation is selected and output width is less than the input width.  xl_area=[6 0 0 12 0 0 0]  block_version=VER_STRING_GOES_HERE
  Mux : xbsIndex_r4/Mux  inputs=2  en=off  latency=1  precision=Full  arith_type="Signed  (2's comp)"  n_bits=8  bin_pt=2  quantization=Truncate  overflow=Wrap  dbl_ovrd=off  block_type=mux
      settings: xl_area=[6 11 0 11 0 0 0]  block_version=VER_STRING_GOES_HERE
  Mux1 : xbsIndex_r4/Mux  inputs=2  en=off  latency=1  precision=Full  arith_type="Signed  (2's comp)"  n_bits=8  bin_pt=2  quantization=Truncate  overflow=Wrap  dbl_ovrd=off  block_type=mux
      settings: xl_area=[6 12 0 12 0 0 0]  block_version=VER_STRING_GOES_HERE
  Shift : xbsIndex_r4/Shift  shift_dir=Right  shift_bits=1  en=off  latency=0  precision=User Defined  arith_type="Signed  (2's comp)"  n_bits=10  bin_pt=0  quantization=Truncate  overflow=Wrap  dbl_ovrd=off  block_type=shift
      settings: xl_area=[0 0 0 0 0 0 0]  block_version=VER_STRING_GOES_HERE
  Shift1 : xbsIndex_r4/Shift  shift_dir=Right  shift_bits=2  en=off  latency=0  precision=User Defined  arith_type="Signed  (2's comp)"  n_bits=11  bin_pt=0  quantization=Truncate  overflow=Wrap  dbl_ovrd=off  block_type=shift
      settings: xl_area=[0 0 0 0 0 0 0]  block_version=VER_STRING_GOES_HERE
  H : Outport  OutDataType=sfix(16)  OutScaling=2^0
  L : Outport  Port=2  OutDataType=sfix(16)  OutScaling=2^0
  wires:
  Buffer6/1 -> AddSub4/2
  Buffer2/1 -> AddSub1/1
  Buffer11/1 -> Mux1/1
  Constant2/1 -> Mux1/3
  AddSub2/1 -> Mux1/2
  Mux1/1 -> AddSub3/1
  AddSub4/1 -> [ynM1]
  Buffer14/1 -> L/1
  Buffer13/1 -> H/1
  [xnP1] -> Buffer6/1
  Shift1/1 -> AddSub4/1
  [eol] -> Buffer11/1
  AddSub3/1 -> Shift1/1
  Buffer10/1 -> Mux/1
  [sol] -> Buffer10/1
  Constant1/1 -> Mux/3
  AddSub1/1 -> Mux/2
  Mux/1 -> [yn]
  sol/1 -> [sol]
  Xodd/1 -> Buffer4/1
  Xeven/1 -> Buffer3/1
  [xn] -> Buffer2/1
  Convert2/1 -> Buffer14/1
  Convert1/1 -> Buffer13/1
  [ynM1] -> Convert2/1
  [yn] -> Convert1/1
  [ynM2] -> AddSub2/2
  [yn] -> AddSub2/1
  Buffer1/1 -> [ynM2]
  [yn] -> Buffer1/1
  Buffer5/1 -> [xnM1]
  Buffer3/1 -> [xnP1], Buffer5/1
  [xnP1] -> AddSub/1
  [xnM1] -> AddSub/2
  AddSub/1 -> Shift/1
  Shift/1 -> AddSub1/2
  Constant/1 -> AddSub3/2
  eol/1 -> [eol]
  Buffer4/1 -> [xn]

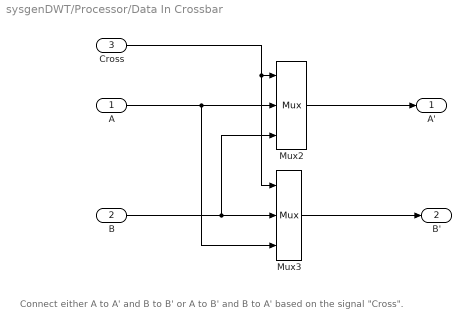
== system sysgenDWT/Processor/Data In Crossbar ==
  note: Connect either A to A' and B to B'
      | or A to B' and B to A' based on
      | the signal "Cross".
  A : Inport  OutDataType=sfix(16)  OutScaling=2^0
  B : Inport  Port=2  OutDataType=sfix(16)  OutScaling=2^0
  Cross : Inport  Port=3  OutDataType=sfix(16)  OutScaling=2^0
  Mux2 : xbsIndex_r4/Mux  inputs=2  en=off  latency=1  precision=Full  arith_type="Signed  (2's comp)"  n_bits=8  bin_pt=2  quantization=Truncate  overflow=Wrap  dbl_ovrd=off  block_type=mux
      settings: xl_area=[5 10 0 10 0 0 0]  block_version=VER_STRING_GOES_HERE
  Mux3 : xbsIndex_r4/Mux  inputs=2  en=off  latency=1  precision=Full  arith_type="Signed  (2's comp)"  n_bits=8  bin_pt=2  quantization=Truncate  overflow=Wrap  dbl_ovrd=off  block_type=mux
      settings: xl_area=[5 10 0 10 0 0 0]  block_version=VER_STRING_GOES_HERE
  A' : Outport  OutDataType=sfix(16)  OutScaling=2^0
  B' : Outport  Port=2  OutDataType=sfix(16)  OutScaling=2^0
  wires:
  Mux2/1 -> A'/1
  Mux3/1 -> B'/1
  A/1 -> Mux2/2, Mux3/3
  B/1 -> Mux3/2, Mux2/3
  Cross/1 -> Mux2/1, Mux3/1

== system sysgenDWT/Processor/Data Out Crossbar ==
  note: Connect either A to A' and B to B'
      | or A to B' and B to A' based on
      | the signal "Cross".
  A : Inport  OutDataType=sfix(16)  OutScaling=2^0
  B : Inport  Port=2  OutDataType=sfix(16)  OutScaling=2^0
  Cross : Inport  Port=3  OutDataType=sfix(16)  OutScaling=2^0
  Mux2 : xbsIndex_r4/Mux  inputs=2  en=off  latency=1  precision=Full  arith_type="Signed  (2's comp)"  n_bits=8  bin_pt=2  quantization=Truncate  overflow=Wrap  dbl_ovrd=off  block_type=mux
      settings: xl_area=[5 10 0 10 0 0 0]  block_version=VER_STRING_GOES_HERE
  Mux3 : xbsIndex_r4/Mux  inputs=2  en=off  latency=1  precision=Full  arith_type="Signed  (2's comp)"  n_bits=8  bin_pt=2  quantization=Truncate  overflow=Wrap  dbl_ovrd=off  block_type=mux
      settings: xl_area=[5 10 0 10 0 0 0]  block_version=VER_STRING_GOES_HERE
  A' : Outport  OutDataType=sfix(16)  OutScaling=2^0
  B' : Outport  Port=2  OutDataType=sfix(16)  OutScaling=2^0
  wires:
  Cross/1 -> Mux3/1, Mux2/1
  B/1 -> Mux2/3, Mux3/2
  A/1 -> Mux3/3, Mux2/2
  Mux3/1 -> B'/1
  Mux2/1 -> A'/1
